simulink model "pendulum_model"  (R2019b)
settings: Solver=VariableStepAuto  StartTime=0.0  StopTime=10.0  RelTol=1e-3
settings Model: Creator=Mike Dermksian  LastModifiedBy=Mike Dermksian
settings DataIOCC: ExternalInput=getinputstruct(op_trim1)  InitialState=getstatestruct(op_trim1)  LoadExternalInput=on  LoadInitialState=on

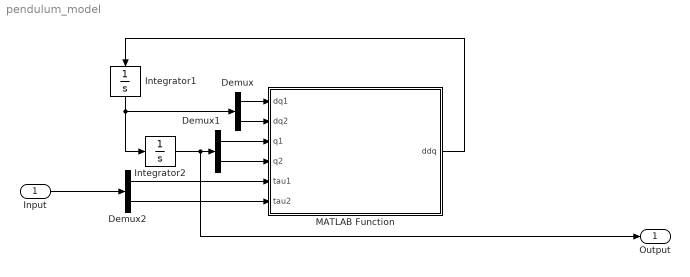
== system pendulum_model ==
  Input : Inport
  Demux : Demux  Outputs=2
  Demux1 : Demux  Outputs=2
  Demux2 : Demux  Outputs=2
  Integrator1 : Integrator  InitialCondition=[0, 0]
  Integrator2 : Integrator  InitialCondition=[pi/2, -pi/2]
  MATLAB Function : MATLAB Function  TreatAsAtomicUnit=on
  Output : Outport
  wires:
  Integrator1/1 -> Demux/1, Integrator2/1
  MATLAB Function/1(ddq) -> Integrator1/1
  Integrator2/1 -> Output/1, Demux1/1
  Demux/1 -> MATLAB Function/1(dq1)
  Demux/2 -> MATLAB Function/2(dq2)
  Demux1/1 -> MATLAB Function/3(q1)
  Demux1/2 -> MATLAB Function/4(q2)
  Demux2/1 -> MATLAB Function/5(tau1)
  Demux2/2 -> MATLAB Function/6(tau2)
  Input/1 -> Demux2/1

== matlab function pendulum_model/MATLAB Function ==
  data: dq1 input; ddq output; dq2 input; q1 input; q2 input; tau1 input; tau2 input
function ddq = pendulum_dyn(dq1,dq2,q1,q2,tau1,tau2)
t2 = cos(q1);
t3 = cos(q2);
t4 = sin(q2);
t5 = q1+q2;
t6 = dq1.^2;
t10 = -tau2;
t7 = t3+1.0;
t8 = t3.^2;
t9 = cos(t5);
t11 = t2.*2.0e+1;
t12 = t4.*t6;
t13 = -t11;
t14 = t9.*1.0e+1;
t15 = t8-2.0;
t16 = -t14;
t17 = 1.0./t15;
t18 = t10+t12+t14;
ddq = [-t17.*(t13+t16+tau1+dq2.*t4.*(dq1+dq2)+dq1.*dq2.*t4)-t7.*t17.*t18;t7.*t17.*(t13+t16+tau1+dq2.^2.*t4+dq1.*dq2.*t4.*2.0)+t17.*t18.*(t7.*2.0+1.0)];
